simulink model "old_quest"  (R2025a)
settings: Solver=VariableStepAuto  StartTime=0.0  StopTime=10.0  RelTol=1e-3
undefined symbols (not defined in the file): weight_B, weight_S
libraries: vrlib x4
settings Model: Creator=procyon  LastModifiedBy=procyon

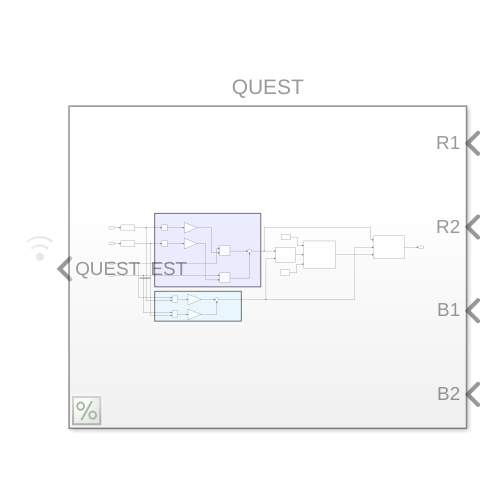
[thumbnail: Simulink's stored preview of the top-level diagram]
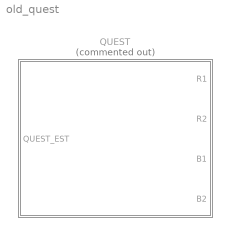
== system old_quest ==
  QUEST : Subsystem  Commented=on

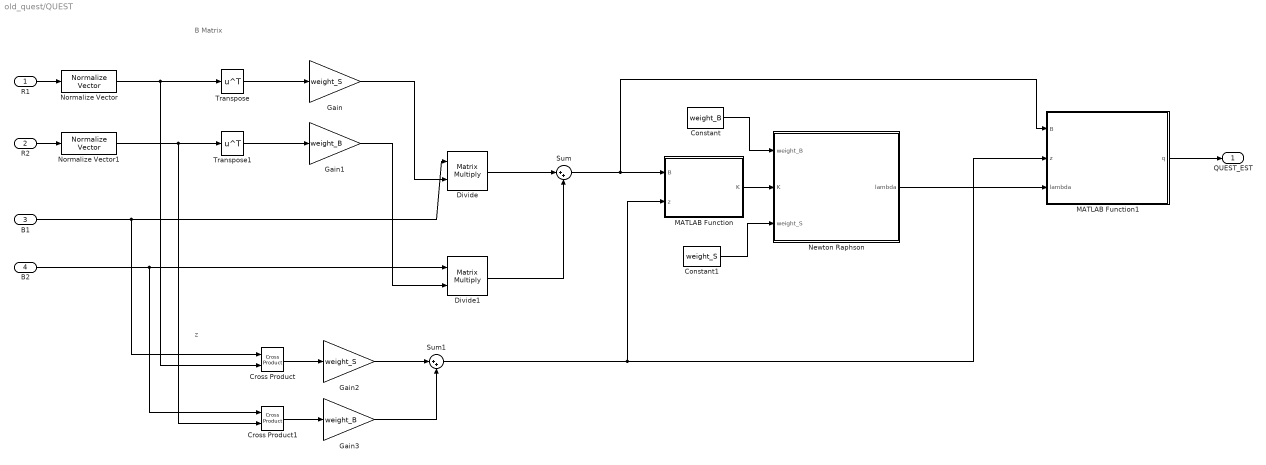
== system old_quest/QUEST ==
  note: z
  note: B Matrix
  R1 : Inport
  R2 : Inport  Port=2
  B1 : Inport  Port=3
  B2 : Inport  Port=4
  Constant : Constant  Value=weight_B
  Constant1 : Constant  Value=weight_S
  Cross Product : vrlib/Utilities/Cross Product
  Cross Product1 : vrlib/Utilities/Cross Product
  Divide : Product  Inputs=**  Multiplication=Matrix(*)
  Divide1 : Product  Inputs=**  Multiplication=Matrix(*)
  Gain : Gain  Gain=weight_S
  Gain1 : Gain  Gain=weight_B
  Gain2 : Gain  Gain=weight_S
  Gain3 : Gain  Gain=weight_B
  MATLAB Function : MATLAB Function  TreatAsAtomicUnit=on
  MATLAB Function1 : MATLAB Function  TreatAsAtomicUnit=on
  Newton Raphson : MATLAB Function  TreatAsAtomicUnit=on
  Normalize Vector : vrlib/Utilities/Normalize Vector  maxzero=0
  Normalize Vector1 : vrlib/Utilities/Normalize Vector  maxzero=0
  Sum : Sum  Inputs=|++
  Sum1 : Sum  Inputs=|++
  Transpose : Math  Operator=transpose
  Transpose1 : Math  Operator=transpose
  QUEST_EST : Outport
  wires:
  R1/1 -> Normalize Vector/1
  R2/1 -> Normalize Vector1/1
  Normalize Vector/1 -> Cross Product/2, Transpose/1
  Transpose/1 -> Gain/1
  Transpose1/1 -> Gain1/1
  Divide/1 -> Sum/1
  Divide1/1 -> Sum/2
  Gain1/1 -> Divide1/2
  Gain/1 -> Divide/2
  B1/1 -> Cross Product/1, Divide/1
  Cross Product/1 -> Gain2/1
  Normalize Vector1/1 -> Cross Product1/2, Transpose1/1
  Cross Product1/1 -> Gain3/1
  B2/1 -> Cross Product1/1, Divide1/1
  Gain2/1 -> Sum1/1
  Gain3/1 -> Sum1/2
  Sum/1 -> MATLAB Function/1(B), MATLAB Function1/1(B)
  Sum1/1 -> MATLAB Function1/2(z), MATLAB Function/2(z)
  MATLAB Function/1(K) -> Newton Raphson/2(K)
  Constant/1 -> Newton Raphson/1(weight_B)
  Constant1/1 -> Newton Raphson/3(weight_S)
  Newton Raphson/1(lambda) -> MATLAB Function1/3(lambda)
  MATLAB Function1/1(q) -> QUEST_EST/1

== matlab function old_quest/QUEST/MATLAB Function ==
  data: B input; K output; z input
function K = K_B(B, z)
% K(B) = [ B + B.' - (trace(B))*I3,  z ;
%          z.',                     trace(B) ]

    trB = trace(B);
    S   = B + B.';
    z   = z(:);              % ensure 3x1

    K = [ S - trB*eye(3), z ;
          z.',             trB ];
end

== matlab function old_quest/QUEST/MATLAB Function1 ==
  data: B input; q output; z input; lambda input
function q = quest_qopt(B, z, lambda)
% q_opt from B, z, lambda where rho = lambda + tr(B)
% q = [q1;q2;q3;q4] (normalized; flips sign to make q4 >= 0)

    % checks
    if ~isequal(size(B),[3 3]); error('B must be 3x3'); end
    z = z(:);
    if ~isequal(size(z),[3 1]); error('z must be 3x1'); end

    trB = trace(B);
    S   = B + B.';
    rho = lambda + trB;
    A   = rho*eye(3) - S;

    % adj(A) via cofactors (works even if A is singular)
    a=A(1,1); b=A(1,2); c=A(1,3);
    d=A(2,1); e=A(2,2); f=A(2,3);
    g=A(3,1); h=A(3,2); i=A(3,3);
    adjA = [ e*i - f*h,  c*h - b*i,  b*f - c*e;
             f*g - d*i,  a*i - c*g,  c*d - a*f;
             d*h - e*g,  b*g - a*h,  a*e - b*d ];

    top  = adjA * z;
    bot  = det(A);

    q = [top; bot];
    n = norm(q);
    if ~isfinite(n) || n == 0
        error('Degenerate inputs');
    end
    q = q / n;
    if q(4) < 0, q = -q; end

    q = [q(4); q(1:3)];
    
end

== matlab function old_quest/QUEST/Newton Raphson ==
  data: weight_B input; lambda output; K input; weight_S input
function lambda = fcn(weight_B, K, weight_S)
    % Newton–Raphson no polinômio característico de K
    coeffs     = poly(K);
    coeffs_der = polyder(coeffs);

    lambda = weight_B + weight_S;   % chute inicial
    max_iter  = 100;
    tol_f     = 1e-12;              % tolerância em f(lambda)
    tol_step  = 1e-12;              % tolerância no passo relativo

    for i = 1:max_iter
        f  = polyval(coeffs, lambda);
        fp = polyval(coeffs_der, lambda);

        if ~isfinite(fp) || fp == 0
            % Derivada zero/NaN: evite divisão por zero
            break
        end

        step   = f / fp;
        lambda_new = lambda - step;

        % Critérios de parada: valor da função e tamanho do passo
        if abs(f) < tol_f || abs(lambda_new - lambda) <= tol_step*(1+abs(lambda))
            lambda = lambda_new;
            break
        end

        lambda = lambda_new;
    end
end
